simulink model "Zadanie"  (Simulink 4.00)
settings: Solver=ode45  StartTime=0.0  StopTime=10.0  RelTol=1e-3
settings Model: LastModifiedBy=user

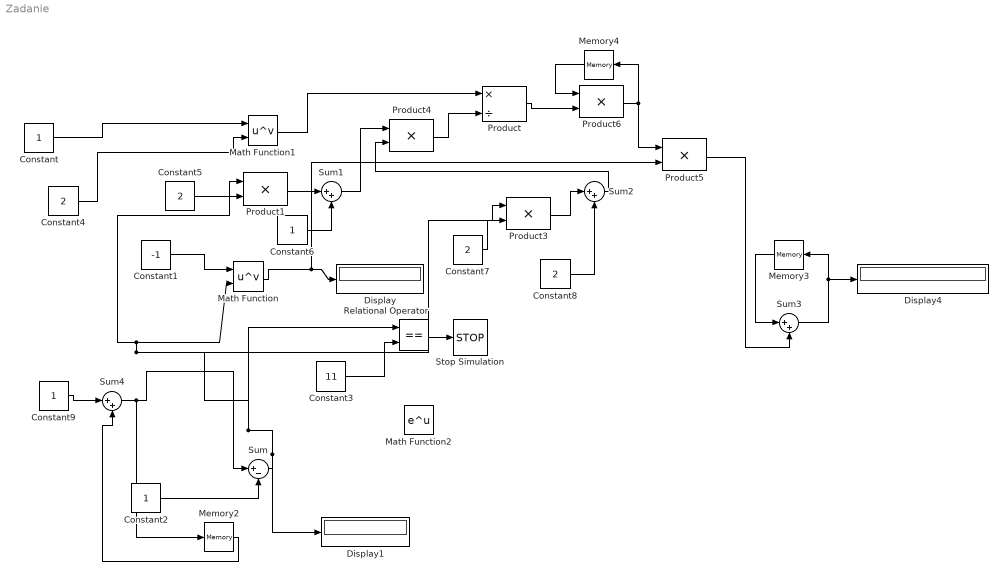
== system Zadanie ==
  Constant{,2,6,9} (4 alike) : Constant  Value=1
  Constant1 : Constant  Value=-1
  Constant3 : Constant  Value=11
  Constant{4..5,7..8} (4 alike) : Constant  Value=2
  Display : Display
      settings: Format=short
  Display1 : Display
      settings: Format=short
  Display4 : Display
  Math Function : Math  Operator=pow  OutputSignalType=auto
  Math Function1 : Math  Operator=pow  OutputSignalType=auto
  Math Function2 : Math  Operator=exp  OutputSignalType=auto
  Memory2 : Memory  X0=0  InheritSampleTime=off
      settings: RTWStateStorageClass=Auto
  Memory3 : Memory  Orientation=left  X0=1  InheritSampleTime=off
      settings: RTWStateStorageClass=Auto
  Memory4 : Memory  Orientation=left  X0=0  InheritSampleTime=off
      settings: RTWStateStorageClass=Auto
  Product : Product  Inputs=*/  Multiplication=Element-wise(.*)  SaturateOnIntegerOverflow=on
  Product1 : Product  Inputs=2  Multiplication=Element-wise(.*)  SaturateOnIntegerOverflow=on
  Product3 : Product  Inputs=2  Multiplication=Element-wise(.*)  SaturateOnIntegerOverflow=on
  Product4 : Product  Inputs=2  Multiplication=Element-wise(.*)  SaturateOnIntegerOverflow=on
  Product5 : Product  Inputs=**  Multiplication=Element-wise(.*)  SaturateOnIntegerOverflow=on
  Product6 : Product  Inputs=**  Multiplication=Element-wise(.*)  SaturateOnIntegerOverflow=on
  Relational Operator : RelationalOperator  Operator===
  Stop Simulation : Stop
  Sum : Sum  Inputs=|+-  SaturateOnIntegerOverflow=on
  Sum{1..4} (4 alike) : Sum  Inputs=|++  SaturateOnIntegerOverflow=on
  wires:
  Constant1/1 -> Math Function/1
  Math Function/1 -> Display/1, Product5/2
  Constant2/1 -> Sum/2
  Memory2/1 -> Sum4/2
  Sum/1 -> Relational Operator/1, Math Function/2, Product1/1, Product3/1, Display1/1
  Relational Operator/1 -> Stop Simulation/1
  Constant3/1 -> Relational Operator/2
  Constant/1 -> Math Function1/1
  Constant4/1 -> Math Function1/2
  Math Function1/1 -> Product/1
  Constant5/1 -> Product1/2
  Constant6/1 -> Sum1/2
  Product1/1 -> Sum1/1
  Constant7/1 -> Product3/2
  Constant8/1 -> Sum2/2
  Product3/1 -> Sum2/1
  Sum2/1 -> Product4/2
  Sum1/1 -> Product4/1
  Product4/1 -> Product/2
  Memory3/1 -> Sum3/1
  Sum3/1 -> Memory3/1, Display4/1
  Product5/1 -> Sum3/2
  Product/1 -> Product6/2
  Memory4/1 -> Product6/1
  Product6/1 -> Memory4/1, Product5/1
  Constant9/1 -> Sum4/1
  Sum4/1 -> Memory2/1, Sum/1
